simulink model "FlSys_FlConsTot"  (R2016b)
settings: configuration reference "CodeGenConfigSet" (kept outside this file)
undefined symbols (not defined in the file or in its folder): EngState_conv, FlSys_FlConsTot_DT
libraries: CXLib x1
settings Model: Creator=Administrator  LastModifiedBy=yushengzhou
settings ConfigSetRef: SourceLocation=Base Workspace

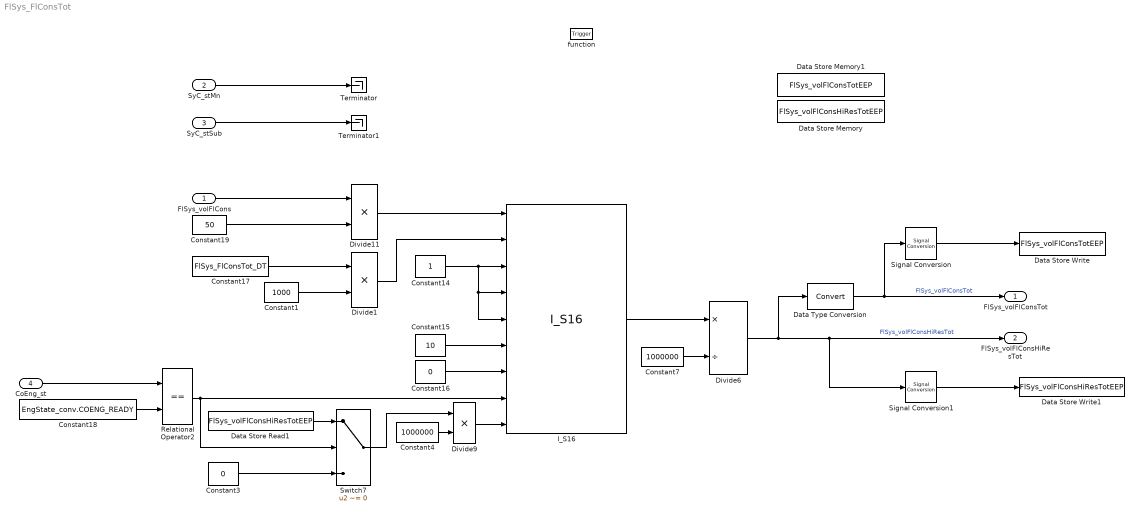
== system FlSys_FlConsTot ==
  FlSys_volFlCons : Inport  Tag=ul/20ms  Description=absolute fuel consumption in ul/DT  OutMin=-2147483648  OutMax=2147483647  OutDataTypeStr=FlConsum_ul_20ms
  SyC_stMn : Inport  Description=Current system/ECU state  Port=2  OutDataTypeStr=Enum: SysExeState_conv
  SyC_stSub : Inport  Description=Current system/ECU sub-state  Port=3  OutDataTypeStr=Enum: SubSysExeState_conv
  CoEng_st : Inport  Description=Engine coordinator state  Port=4  OutDataTypeStr=Enum: EngState_conv
  function : TriggerPort  TriggerType=function-call  VariantControl=Variant
  Constant1 : Constant  Value=1000  OutDataTypeStr=uint16
  Constant14 : Constant  OutDataTypeStr=Inherit: Inherit via back propagation
  Constant15 : Constant  Value=10  OutDataTypeStr=Inherit: Inherit via back propagation
  Constant16 : Constant  Value=0  OutDataTypeStr=Inherit: Inherit via back propagation
  Constant17 : Constant  Value=FlSys_FlConsTot_DT
  Constant18 : Constant  Value=EngState_conv.COENG_READY
  Constant19 : Constant  Value=50  OutDataTypeStr=uint8
  Constant3 : Constant  Value=0  OutDataTypeStr=Inherit: Inherit via back propagation
  Constant4 : Constant  Value=1000000  OutDataTypeStr=int32
  Constant7 : Constant  Value=1000000  OutDataTypeStr=int32
  Data Store Memory : DataStoreMemory  DataStoreName=FlSys_volFlConsHiResTotEEP  ReadBeforeWriteMsg=warning  WriteAfterWriteMsg=warning  WriteAfterReadMsg=warning  ShowAdditionalParam=off
  Data Store Memory1 : DataStoreMemory  DataStoreName=FlSys_volFlConsTotEEP  ReadBeforeWriteMsg=warning  WriteAfterWriteMsg=warning  WriteAfterReadMsg=warning  ShowAdditionalParam=off
  Data Store Read1 : DataStoreRead  DataStoreName=FlSys_volFlConsHiResTotEEP
  Data Store Write : DataStoreWrite  DataStoreName=FlSys_volFlConsTotEEP
  Data Store Write1 : DataStoreWrite  DataStoreName=FlSys_volFlConsHiResTotEEP
  Data Type Conversion : DataTypeConversion
  Divide1 : Product  Inputs=**  OutDataTypeStr=uint32  SaturateOnIntegerOverflow=on
  Divide11 : Product  Inputs=**  OutDataTypeStr=int32  SaturateOnIntegerOverflow=on
  Divide6 : Product  Inputs=*/  OutDataTypeStr=Inherit: Inherit via back propagation  RndMeth=Round  SaturateOnIntegerOverflow=on
  Divide9 : Product  Inputs=**  OutDataTypeStr=uint32  RndMeth=Round  SaturateOnIntegerOverflow=on
  I_S16 : CXLib/I_S16
  Relational Operator2 : RelationalOperator  Operator===  OutDataTypeStr=boolean  RndMeth=Simplest  InputSameDT=on
  Signal Conversion : SignalConversion  OverrideOpt=off
  Signal Conversion1 : SignalConversion  OverrideOpt=off
  Switch7 : Switch  Criteria=u2 ~= 0  SaturateOnIntegerOverflow=on  InputSameDT=on
  Terminator : Terminator
  Terminator1 : Terminator
  FlSys_volFlConsTot : Outport  Tag=L  Description=fuel consumption per driving cycle [ul] (only torque relevant injection quantity)  OutMin=0  OutMax=2147483647  OutDataTypeStr=Fl_Half_L
  FlSys_volFlConsHiResTot : Outport  Tag=L  Description=TotalFuelConsumption having higher resolution  Port=2  OutMin=0  OutMax=4294967  OutDataTypeStr=FlConsum_L
  wires:
  SyC_stMn/1 -> Terminator/1
  SyC_stSub/1 -> Terminator1/1
  FlSys_volFlCons/1 -> Divide11/1
  Relational Operator2/1 -> I_S16/8, Switch7/2
  Data Store Read1/1 -> Switch7/1
  Switch7/1 -> Divide9/1
  Constant14/1 -> I_S16/5, I_S16/4, I_S16/3
  Constant15/1 -> I_S16/6
  Constant16/1 -> I_S16/7
  Constant3/1 -> Switch7/3
  Divide6/1 -> Signal Conversion1/1, FlSys_volFlConsHiResTot/1, Data Type Conversion/1  "FlSys_volFlConsHiResTot"
  Constant7/1 -> Divide6/2
  I_S16/1 -> Divide6/1
  Data Type Conversion/1 -> Signal Conversion/1, FlSys_volFlConsTot/1  "FlSys_volFlConsTot"
  Signal Conversion1/1 -> Data Store Write1/1
  Signal Conversion/1 -> Data Store Write/1
  Constant18/1 -> Relational Operator2/2
  CoEng_st/1 -> Relational Operator2/1
  Constant4/1 -> Divide9/2
  Divide9/1 -> I_S16/9
  Constant19/1 -> Divide11/2
  Divide11/1 -> I_S16/1
  Constant17/1 -> Divide1/1
  Constant1/1 -> Divide1/2
  Divide1/1 -> I_S16/2
